simulink model "square_wave_gen"  (R2018b)
settings: Solver=VariableStepAuto  StartTime=0.0  StopTime=5e-2  RelTol=1e-3
settings Model: Creator=sangh  LastModifiedBy=sangh

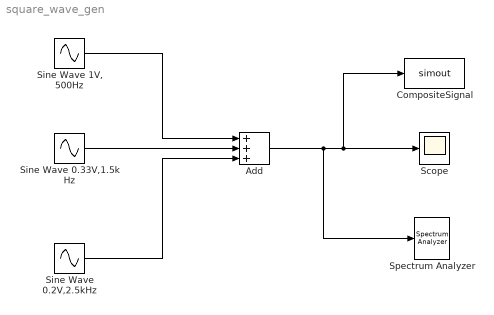
== system square_wave_gen ==
  Add : Sum  Inputs=+++
  CompositeSignal : ToWorkspace  VariableName=simout  SaveFormat=Timeseries  SampleTime=-1
  Scope : Scope
  Sine Wave 0.2V,2.5kHz : Sin  Amplitude=1/5  Frequency=2*pi*2.5e3  SampleTime=0.25e-6
  Sine Wave 0.33V,1.5kHz : Sin  Amplitude=1/3  Frequency=2*pi*1500  SampleTime=0.25e-6
  "Sine Wave 1V, 500Hz" : Sin  Frequency=2*pi*500  SampleTime=0.25e-6
  Spectrum Analyzer : SpectrumAnalyzer
  wires:
  "Sine Wave 1V, 500Hz"/1 -> Add/1
  Sine Wave 0.33V,1.5kHz/1 -> Add/2
  Sine Wave 0.2V,2.5kHz/1 -> Add/3
  Add/1 -> Spectrum Analyzer/1, CompositeSignal/1, Scope/1
